simulink model "non-lin_model"  (R2019a)
settings: Solver=VariableStepAuto  StartTime=0.0  StopTime=10  RelTol=1e-3
values from neighbouring files (symbols this model uses):
  g = 9.80665    [drone.m]    (also in step-af-drone.m = -150*(1+0.001*s)/s)
undefined symbols (not defined in the file or in its folder): b, d, Ir, Ix, Iy, Iz, l, m
settings Model: Creator=Hillerup  LastModifiedBy=Hillerup

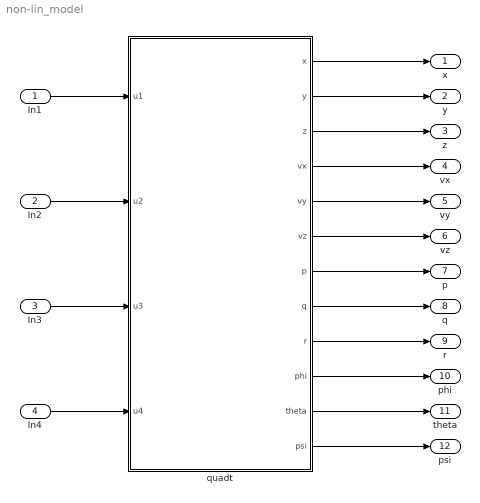
== system non-lin_model ==
  In1 : Inport
  In2 : Inport  Port=2
  In3 : Inport  Port=3
  In4 : Inport  Port=4
  quadt : Subsystem
  "x " : Outport
  y : Outport  Port=2
  z : Outport  Port=3
  vx : Outport  Port=4
  vy : Outport  Port=5
  vz : Outport  Port=6
  p : Outport  Port=7
  q : Outport  Port=8
  r : Outport  Port=9
  phi : Outport  Port=10
  theta : Outport  Port=11
  psi : Outport  Port=12
  wires:
  quadt/1("x ") -> "x "/1
  quadt/2(y) -> y/1
  quadt/3(z) -> z/1
  quadt/4(vx) -> vx/1
  quadt/5(vy) -> vy/1
  quadt/6(vz) -> vz/1
  quadt/8(q) -> q/1
  quadt/9(r) -> r/1
  quadt/10(phi) -> phi/1
  quadt/11(theta) -> theta/1
  quadt/12(psi) -> psi/1
  quadt/7(p) -> p/1
  In1/1 -> quadt/1(u1)
  In2/1 -> quadt/2(u2)
  In3/1 -> quadt/3(u3)
  In4/1 -> quadt/4(u4)

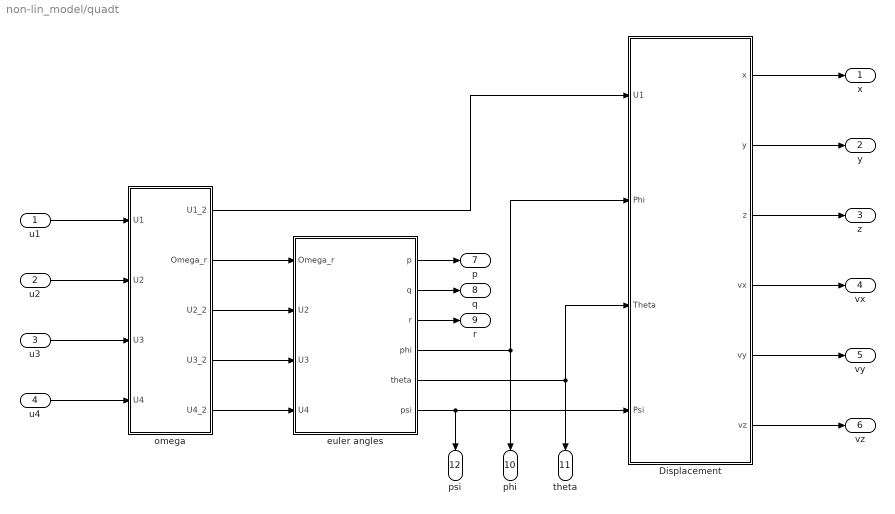
== system non-lin_model/quadt ==
  u1 : Inport
  u2 : Inport  Port=2
  u3 : Inport  Port=3
  u4 : Inport  Port=4
  Displacement : Subsystem
  euler angles : Subsystem
  omega : Subsystem
  "x " : Outport
  y : Outport  Port=2
  z : Outport  Port=3
  vx : Outport  Port=4
  vy : Outport  Port=5
  vz : Outport  Port=6
  p : Outport  Port=7
  q : Outport  Port=8
  r : Outport  Port=9
  phi : Outport  Port=10
  theta : Outport  Port=11
  psi : Outport  Port=12
  wires:
  euler angles/1(p) -> p/1
  euler angles/5(theta) -> Displacement/3(Theta), theta/1
  Displacement/1(x) -> "x "/1
  Displacement/6(vz) -> vz/1
  Displacement/5(vy) -> vy/1
  euler angles/4(phi) -> Displacement/2(Phi), phi/1
  euler angles/6(psi) -> Displacement/4(Psi), psi/1
  Displacement/2(y) -> y/1
  Displacement/3(z) -> z/1
  Displacement/4(vx) -> vx/1
  euler angles/2(q) -> q/1
  euler angles/3(r) -> r/1
  u1/1 -> omega/1(U1)
  u2/1 -> omega/2(U2)
  u3/1 -> omega/3(U3)
  u4/1 -> omega/4(U4)
  omega/1(U1_2) -> Displacement/1(U1)
  omega/2(Omega_r) -> euler angles/1(Omega_r)
  omega/3(U2_2) -> euler angles/2(U2)
  omega/4(U3_2) -> euler angles/3(U3)
  omega/5(U4_2) -> euler angles/4(U4)

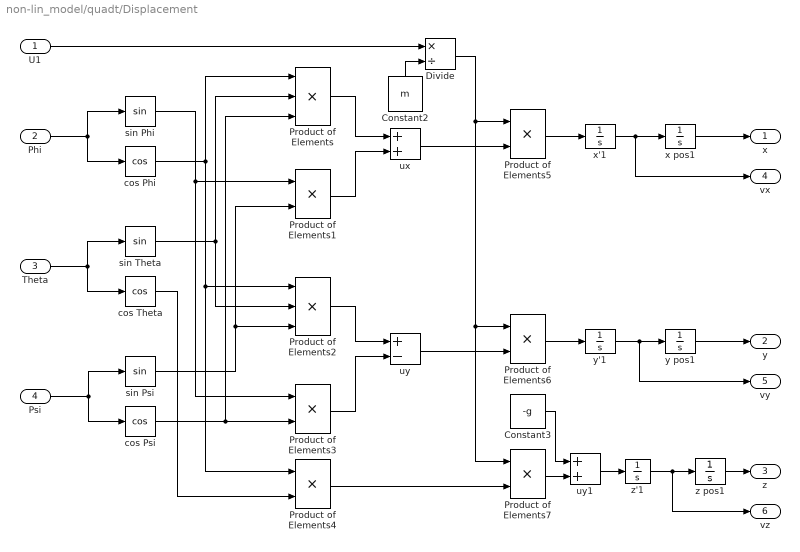
== system non-lin_model/quadt/Displacement ==
  U1 : Inport
  Phi : Inport  Port=2
  Theta : Inport  Port=3
  Psi : Inport  Port=4
  Constant2 : Constant  Value=m
  Constant3 : Constant  Value=-g
  Divide : Product  Inputs=*/
  Product of Elements : Product  Inputs=3
  Product of Elements{1,3..7} (6 alike) : Product
  Product of Elements2 : Product  Inputs=3
  cos Phi : Trigonometry  Operator=cos
  cos Psi : Trigonometry  Operator=cos
  cos Theta : Trigonometry  Operator=cos
  sin Phi : Trigonometry
  sin Psi : Trigonometry
  sin Theta : Trigonometry
  ux : Sum
  uy : Sum  Inputs=+-
  uy1 : Sum
  x pos1 : Integrator
  x'1 : Integrator
  y pos1 : Integrator
  y'1 : Integrator
  z pos1 : Integrator
  z'1 : Integrator
  x : Outport
  y : Outport  Port=2
  z : Outport  Port=3
  vx : Outport  Port=4
  vy : Outport  Port=5
  vz : Outport  Port=6
  wires:
  uy1/1 -> z'1/1
  y pos1/1 -> y/1
  Constant3/1 -> uy1/1
  x pos1/1 -> x/1
  z'1/1 -> vz/1, z pos1/1
  cos Theta/1 -> Product of Elements4/2
  Product of Elements5/1 -> x'1/1
  Constant2/1 -> Divide/2
  Product of Elements/1 -> ux/1
  y'1/1 -> y pos1/1, vy/1
  sin Psi/1 -> Product of Elements1/2, Product of Elements2/3
  Product of Elements1/1 -> ux/2
  Psi/1 -> sin Psi/1, cos Psi/1
  cos Phi/1 -> Product of Elements/1, Product of Elements2/1, Product of Elements4/1
  Product of Elements3/1 -> uy/2
  uy/1 -> Product of Elements6/2
  Product of Elements2/1 -> uy/1
  Divide/1 -> Product of Elements5/1, Product of Elements6/1, Product of Elements7/1
  ux/1 -> Product of Elements5/2
  cos Psi/1 -> Product of Elements/3, Product of Elements3/2
  sin Phi/1 -> Product of Elements1/1, Product of Elements3/1
  Product of Elements7/1 -> uy1/2
  Product of Elements6/1 -> y'1/1
  Theta/1 -> sin Theta/1, cos Theta/1
  x'1/1 -> vx/1, x pos1/1
  Phi/1 -> sin Phi/1, cos Phi/1
  Product of Elements4/1 -> Product of Elements7/2
  sin Theta/1 -> Product of Elements/2, Product of Elements2/2
  z pos1/1 -> z/1
  U1/1 -> Divide/1

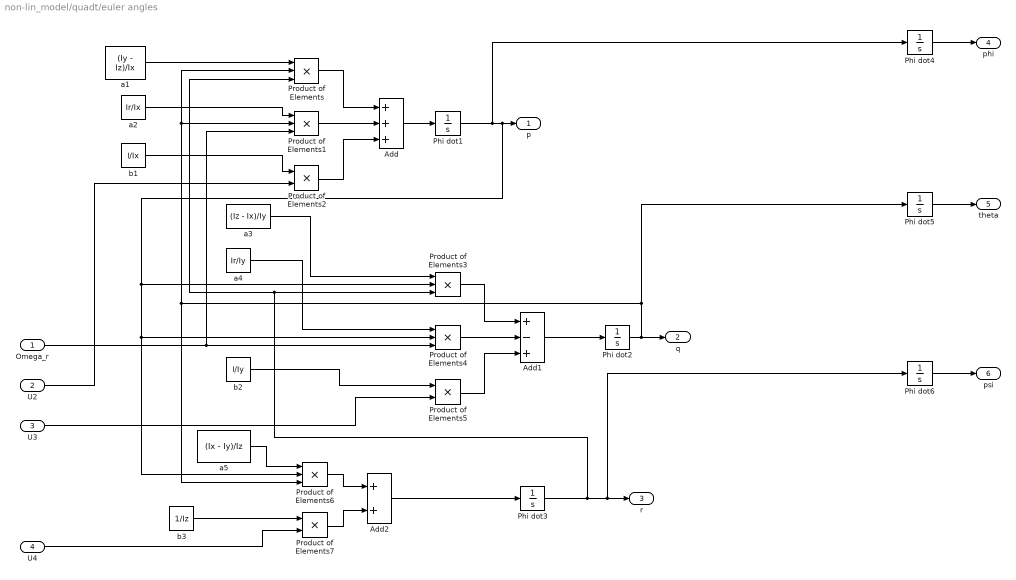
== system non-lin_model/quadt/euler angles ==
  Omega_r : Inport
  U2 : Inport  Port=2
  U3 : Inport  Port=3
  U4 : Inport  Port=4
  Add : Sum  Inputs=+++
  Add1 : Sum  Inputs=+-+
  Add2 : Sum
  Phi dot{1..6} (6 alike) : Integrator
  Product of Elements{,1,3..4,6} (5 alike) : Product  Inputs=3
  Product of Elements2 : Product
  Product of Elements5 : Product
  Product of Elements7 : Product
  a1 : Constant  Value=(Iy - Iz)/Ix
  a2 : Constant  Value=Ir/Ix
  a3 : Constant  Value=(Iz - Ix)/Iy
  a4 : Constant  Value=Ir/Iy
  a5 : Constant  Value=(Ix - Iy)/Iz
  b1 : Constant  Value=l/Ix
  b2 : Constant  Value=l/Iy
  b3 : Constant  Value=1/Iz
  p : Outport
  q : Outport  Port=2
  r : Outport  Port=3
  phi : Outport  Port=4
  theta : Outport  Port=5
  psi : Outport  Port=6
  wires:
  Phi dot2/1 -> q/1, Phi dot5/1, Product of Elements/2, Product of Elements1/2, Product of Elements6/3
  Product of Elements2/1 -> Add/3
  Omega_r/1 -> Product of Elements1/3, Product of Elements4/3
  Product of Elements1/1 -> Add/2
  Product of Elements4/1 -> Add1/2
  a4/1 -> Product of Elements4/1
  b2/1 -> Product of Elements5/1
  a2/1 -> Product of Elements1/1
  Product of Elements/1 -> Add/1
  Product of Elements3/1 -> Add1/1
  a1/1 -> Product of Elements/1
  b1/1 -> Product of Elements2/1
  a5/1 -> Product of Elements6/1
  U2/1 -> Product of Elements2/2
  U3/1 -> Product of Elements5/2
  Product of Elements6/1 -> Add2/1
  Product of Elements7/1 -> Add2/2
  U4/1 -> Product of Elements7/2
  b3/1 -> Product of Elements7/1
  Product of Elements5/1 -> Add1/3
  a3/1 -> Product of Elements3/1
  Add1/1 -> Phi dot2/1
  Add2/1 -> Phi dot3/1
  Add/1 -> Phi dot1/1
  Phi dot1/1 -> Phi dot4/1, Product of Elements3/2, Product of Elements4/2, Product of Elements6/2, p/1
  Phi dot6/1 -> psi/1
  Phi dot5/1 -> theta/1
  Phi dot4/1 -> phi/1
  Phi dot3/1 -> Phi dot6/1, r/1, Product of Elements/3, Product of Elements3/3

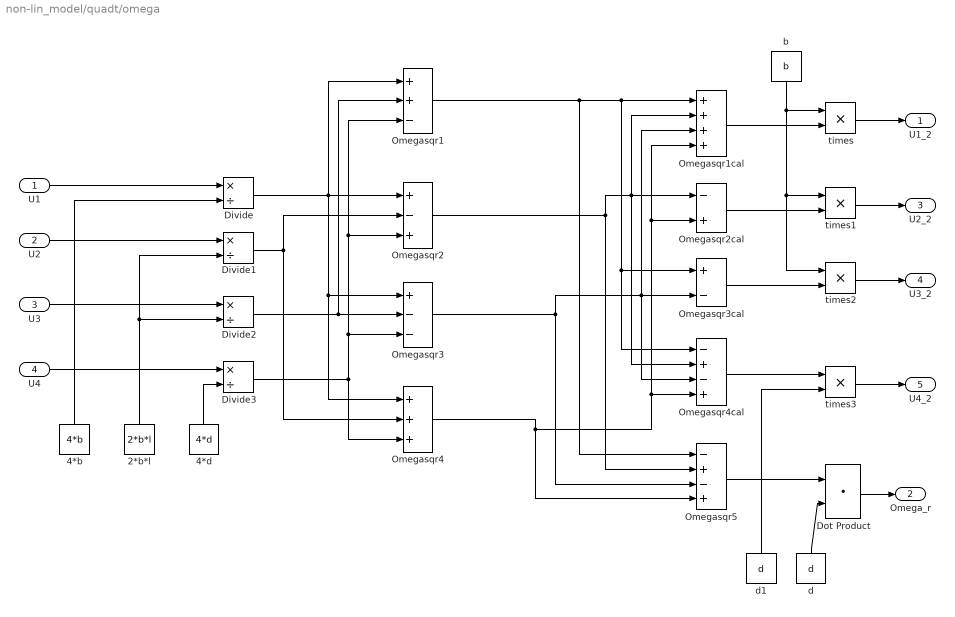
== system non-lin_model/quadt/omega ==
  U1 : Inport
  U2 : Inport  Port=2
  U3 : Inport  Port=3
  U4 : Inport  Port=4
  2*b*l : Constant  Value=2*b*l
  4*b : Constant  Value=4*b
  4*d : Constant  Value=4*d
  Divide{,1..3} (4 alike) : Product  Inputs=*/
  Dot Product : DotProduct  InputSameDT=on  OutDataTypeStr=Inherit: Inherit via internal rule
  Omegasqr1 : Sum  Inputs=++-
  Omegasqr1cal : Sum  Inputs=++++
  Omegasqr2 : Sum  Inputs=+-+
  Omegasqr2cal : Sum  Inputs=-+
  Omegasqr3 : Sum  Inputs=+--
  Omegasqr3cal : Sum  Inputs=+-
  Omegasqr4 : Sum  Inputs=+++
  Omegasqr4cal : Sum  Inputs=-+-+
  Omegasqr5 : Sum  Inputs=-+-+
  b : Constant  Value=b
  d : Constant  Value=d
  d1 : Constant  Value=d
  times{,1..3} (4 alike) : Product  Inputs=**
  U1_2 : Outport
  Omega_r : Outport  Port=2
  U2_2 : Outport  Port=3
  U3_2 : Outport  Port=4
  U4_2 : Outport  Port=5
  wires:
  U1/1 -> Divide/1
  4*b/1 -> Divide/2
  U2/1 -> Divide1/1
  2*b*l/1 -> Divide1/2, Divide2/2
  U3/1 -> Divide2/1
  U4/1 -> Divide3/1
  4*d/1 -> Divide3/2
  Divide/1 -> Omegasqr1/1, Omegasqr4/1, Omegasqr3/1, Omegasqr2/1
  Divide2/1 -> Omegasqr1/2, Omegasqr3/2
  Divide3/1 -> Omegasqr1/3, Omegasqr2/3, Omegasqr3/3, Omegasqr4/3
  Divide1/1 -> Omegasqr2/2, Omegasqr4/2
  Omegasqr5/1 -> Dot Product/1
  Dot Product/1 -> Omega_r/1
  d/1 -> Dot Product/2
  b/1 -> times/1, times1/1, times2/1
  Omegasqr1cal/1 -> times/2
  Omegasqr2cal/1 -> times1/2
  Omegasqr3cal/1 -> times2/2
  Omegasqr4cal/1 -> times3/1
  d1/1 -> times3/2
  times/1 -> U1_2/1
  times1/1 -> U2_2/1
  times3/1 -> U4_2/1
  times2/1 -> U3_2/1
  Omegasqr1/1 -> Omegasqr3cal/1, Omegasqr4cal/1, Omegasqr1cal/1, Omegasqr5/1
  Omegasqr2/1 -> Omegasqr1cal/2, Omegasqr2cal/1, Omegasqr4cal/2, Omegasqr5/2
  Omegasqr3/1 -> Omegasqr1cal/3, Omegasqr3cal/2, Omegasqr4cal/3, Omegasqr5/3
  Omegasqr4/1 -> Omegasqr5/4, Omegasqr1cal/4, Omegasqr2cal/2, Omegasqr4cal/4
